simulink model "Residual_lab"  (R2023b)
settings: Solver=VariableStepAuto  StartTime=0.0  StopTime=20.0  RelTol=1e-3
values from neighbouring files (symbols this model uses):
  den1 = cell2mat(HY3_N1_D.denominator)    [threeDiskOscillator.m]
  den2 = cell2mat(HY3_N2_D.denominator)    [Question_3.m]    (also in threeDiskOscillator.m; threeDiskOscillator_RIG_template_2023.m)
  num_HU2_N1_D = cell2mat(HU2_N1_D.numerator)    [Question_3.m]    (also in threeDiskOscillator.m; threeDiskOscillator_RIG_template_2023.m)
  num_HY1_N1_D = cell2mat(HY1_N1_D.numerator)    [Question_3.m]    (also in threeDiskOscillator.m; threeDiskOscillator_RIG_template_2023.m)
  num_HY2_N1_D = cell2mat(HY2_N1_D.numerator)    [Question_3.m]    (also in threeDiskOscillator.m; threeDiskOscillator_RIG_template_2023.m)
  num_HY2_N2_D = cell2mat(HY2_N2_D.numerator)    [Question_3.m]    (also in threeDiskOscillator.m; threeDiskOscillator_RIG_template_2023.m)
  num_HY3_N1_D = cell2mat(HY3_N1_D.numerator)    [Question_3.m]    (also in threeDiskOscillator.m; threeDiskOscillator_RIG_template_2023.m)
  num_HY3_N2_D = cell2mat(HY3_N2_D.numerator)    [Question_3.m]    (also in threeDiskOscillator.m; threeDiskOscillator_RIG_template_2023.m)
settings Model: Creator=andre  LastModifiedBy=giova

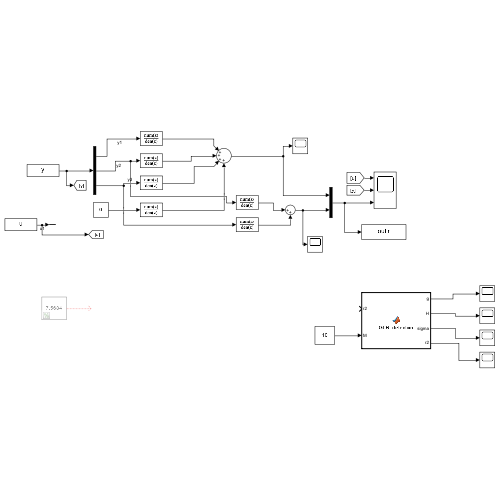
[thumbnail: Simulink's stored preview of the top-level diagram]
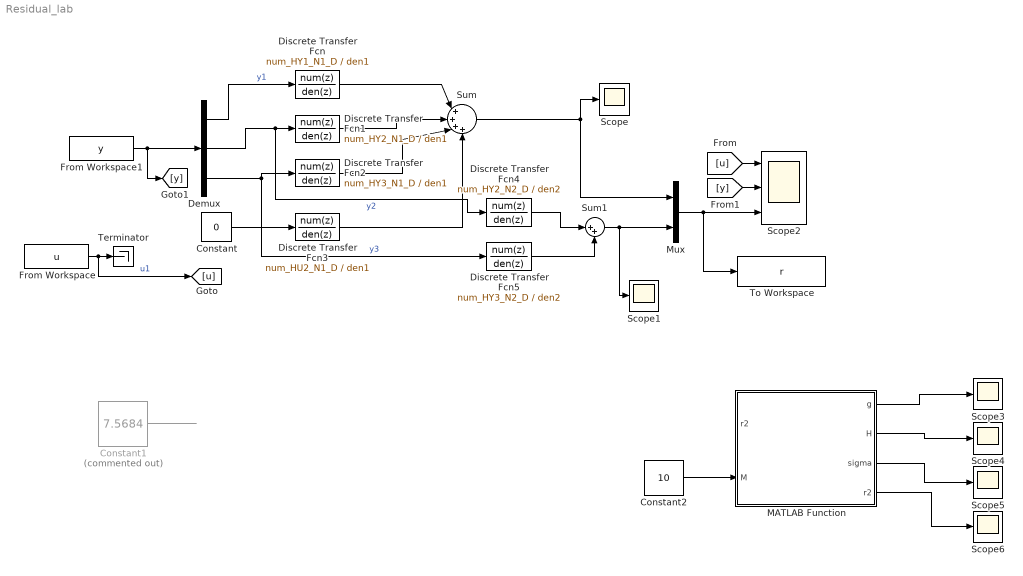
== system Residual_lab ==
  Constant : Constant  Value=0
  Constant1 : Constant  Commented=on  Value=7.5684
  Constant2 : Constant  Value=10
  Demux : Demux  Outputs=3
  Discrete Transfer Fcn : DiscreteTransferFcn  Numerator=num_HY1_N1_D  Denominator=den1
  Discrete Transfer Fcn1 : DiscreteTransferFcn  Numerator=num_HY2_N1_D  Denominator=den1
  Discrete Transfer Fcn2 : DiscreteTransferFcn  Numerator=num_HY3_N1_D  Denominator=den1
  Discrete Transfer Fcn3 : DiscreteTransferFcn  Numerator=num_HU2_N1_D  Denominator=den1
  Discrete Transfer Fcn4 : DiscreteTransferFcn  Numerator=num_HY2_N2_D  Denominator=den2
  Discrete Transfer Fcn5 : DiscreteTransferFcn  Numerator=num_HY3_N2_D  Denominator=den2
  From Workspace : FromWorkspace  VariableName=u
  From Workspace1 : FromWorkspace  VariableName=y  SampleTime=0.004
  MATLAB Function : MATLAB Function  TreatAsAtomicUnit=on
  Mux : Mux  Inputs=2
  Scope{,1,3..6} (6 alike) : Scope
  Scope2 : Scope  NumInputPorts=3
  Sum : Sum  Inputs=|++++
  Sum1 : Sum  Inputs=|++
  Terminator : Terminator
  To Workspace : ToWorkspace  VariableName=r  SaveFormat=Structure With Time  SampleTime=-1
  wires:
  Mux/1 -> To Workspace/1, Scope2/3
  Sum1/1 -> Scope1/1, Mux/2
  Demux/1 -> Discrete Transfer Fcn/1  "y1"
  Discrete Transfer Fcn4/1 -> Sum1/1
  Demux/3 -> Discrete Transfer Fcn5/1, Discrete Transfer Fcn2/1  "y3"
  Demux/2 -> Discrete Transfer Fcn4/1, Discrete Transfer Fcn1/1  "y2"
  Discrete Transfer Fcn5/1 -> Sum1/2
  Sum/1 -> Scope/1, Mux/1
  Discrete Transfer Fcn3/1 -> Sum/4
  Discrete Transfer Fcn1/1 -> Sum/2
  Discrete Transfer Fcn2/1 -> Sum/3
  Discrete Transfer Fcn/1 -> Sum/1
  From Workspace1/1 -> [y], Demux/1
  [y] -> Scope2/2
  [u] -> Scope2/1
  Constant/1 -> Discrete Transfer Fcn3/1
  From Workspace/1 -> [u], Terminator/1  "u1"
  MATLAB Function/1(g) -> Scope3/1
  MATLAB Function/2(H) -> Scope4/1
  Constant1/1 -> ?
  MATLAB Function/4(r2) -> Scope6/1
  MATLAB Function/3(sigma) -> Scope5/1
  Constant2/1 -> MATLAB Function/2(M)

== matlab function Residual_lab/MATLAB Function ==
  data: r2 input; g output; H output; M input; sigma output; r2 output
function [g, H, sigma, r2] = GLR_detection(r2, M)

    % Define parameters
    mu_0 = 0;                   % mean H0
    mu_1 = 0.065;               % mean H1
    sigma = var(r2);             % variance
    % sigma = 0.0011;

    % Calculate g(k)
    g = zeros(size(r2)); 
    for k = M:length(r2)
        maxsum = 0;
        for j = k - M + 1:k
            sumin = (sum(abs(r2(j:k)) - mu_0))^2;
            if sumin > maxsum
                maxsum = sumin;
            end
        end
        g(k) = 1/(2 * sigma * M) * maxsum;
    end
    
    % Calculate function H1 in faulty case
    H = mu_1 * ones(size(r2));

end
